simulink model "R1"  (R2016a)
settings: Solver=VariableStepAuto  StartTime=0.0  StopTime=10.0  RelTol=1e-3
settings Model: Creator=NAD  LastModifiedBy=NAD

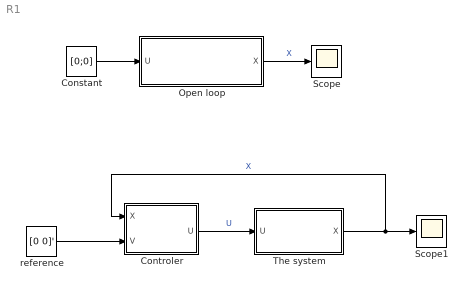
== system R1 ==
  Constant : Constant  Value=[0;0]
  Controler : MATLAB Function  TreatAsAtomicUnit=on
  Open loop : Subsystem
  Scope : Scope
  Scope1 : Scope
  The system : Subsystem
  reference : Constant  Value=[0 0]'
  wires:
  Open loop/1(X) -> Scope/1  "X"
  Constant/1 -> Open loop/1(U)
  The system/1(X) -> Controler/1(X), Scope1/1  "X"
  Controler/1(U) -> The system/1(U)  "U"
  reference/1 -> Controler/2(V)

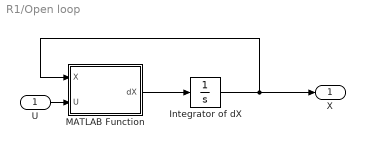
== system R1/Open loop ==
  U : Inport
  Integrator of dX : Integrator  InitialCondition=[1 1 1 1 1 1]
  MATLAB Function : MATLAB Function  TreatAsAtomicUnit=on
  X : Outport
  wires:
  MATLAB Function/1(dX) -> Integrator of dX/1
  U/1 -> MATLAB Function/2(U)
  Integrator of dX/1 -> MATLAB Function/1(X), X/1

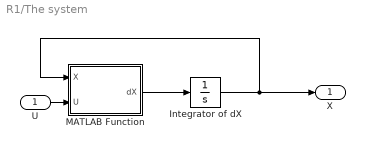
== system R1/The system ==
  U : Inport
  Integrator of dX : Integrator  InitialCondition=[1 1 1 1 1 1]
  MATLAB Function : MATLAB Function  TreatAsAtomicUnit=on
  X : Outport
  wires:
  Integrator of dX/1 -> X/1, MATLAB Function/1(X)
  U/1 -> MATLAB Function/2(U)
  MATLAB Function/1(dX) -> Integrator of dX/1

== matlab function R1/The system/MATLAB Function ==
  data: X input; dX output; U input
function dX = fcn(X,U)
%% Definion of parameters:
x1 = X(1);
x2 = X(2);
x3 = X(3);
x4 = X(4);
x5 = X(5);
x6 = X(6);

u1 = U(1);
u2 = U(2);

e = 1e-3;
%% The system:
dX = [x2
    -sin(x5)*u1 + e*cos(x5)*u2
    x4
    cos(x5)*u1 + e*sin(x5)*u2-1
    x6
    u2 ];

== matlab function R1/Open loop/MATLAB Function ==
  data: X input; dX output; U input
function dX = fcn(X,U)
%% Definion of parameters:
x1 = X(1);
x2 = X(2);
x3 = X(3);
x4 = X(4);
x5 = X(5);
x6 = X(6);

u1 = U(1);
u2 = U(2);

e = 1e-3;
%% The system:
dX = [x2
    -sin(x5)*u1 + e*cos(x5)*u2
    x4
    cos(x5)*u1 + e*sin(x5)*u2-1
    x6
    u2 ];

== matlab function R1/Controler ==
  data: X input; U output; V input
function U = fcn(X,V)
%% Definion of parameters:
x1 = X(1);
x2 = X(2);
x3 = X(3);
x4 = X(4);
x5 = X(5);
x6 = X(6);
e = 1e-3;

%% The feedback:

w0=2;
k1 = w0^2;
k2= 2*w0;

W = [-k1*x1-k2*x2
     -k1*x3-k2*x4] + V ;
 
%% The cintrol: 
B0 = [-sin(x5) e*cos(x5)
       cos(x5) e*sin(x5)];

U = B0\[0;1]+B0\W ;
